simulink model "TestingModels"  (R2021b)
settings: Solver=VariableStepAuto  StartTime=0.0  StopTime=120  FixedStep=1  RelTol=1e-3
libraries: simulink x1
settings Model: Creator=mariodelossantos  LastModifiedBy=mdls3

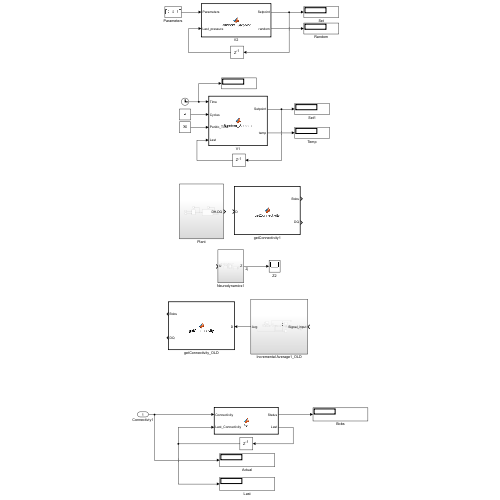
[thumbnail: Simulink's stored preview of the top-level diagram]
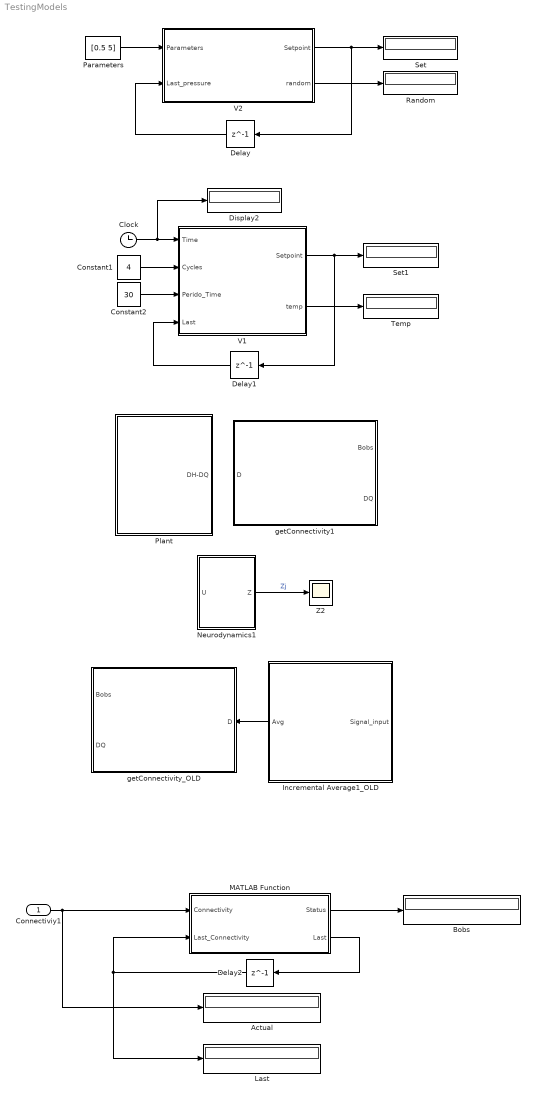
== system TestingModels ==
  Connectiviy1 : Inport
  Actual : Display
  Bobs : Display
  Clock : Clock
  Constant1 : Constant  Value=4
  Constant2 : Constant  Value=30
  Delay : Delay  DelayLength=1  InitialCondition=0
  Delay1 : Delay  DelayLength=1  InitialCondition=0
  Delay2 : Delay  DelayLength=1  InitialCondition=0
  Display2 : Display
  Incremental Average1_OLD : Subsystem
  Last : Display
  MATLAB Function : MATLAB Function  TreatAsAtomicUnit=on
  Neurodynamics1 : Subsystem
  Parameters : Constant  Value=[0.5 5]
  Plant : Subsystem
  Random : Display
  Set : Display
  Set1 : Display
  Temp : Display
  V1 : MATLAB Function  TreatAsAtomicUnit=on
  V2 : MATLAB Function  TreatAsAtomicUnit=on
  Z2 : Scope
  getConnectivity1 : MATLAB Function  TreatAsAtomicUnit=on  SystemSampleTime=0
  getConnectivity_OLD : MATLAB Function  TreatAsAtomicUnit=on  SystemSampleTime=0
  wires:
  Delay/1 -> V2/2(Last_pressure)
  Parameters/1 -> V2/1(Parameters)
  V2/1(Setpoint) -> Delay/1, Set/1
  V2/2(random) -> Random/1
  V1/1(Setpoint) -> Delay1/1, Set1/1
  Delay1/1 -> V1/4(Last)
  Constant1/1 -> V1/2(Cycles)
  Clock/1 -> Display2/1, V1/1(Time)
  Constant2/1 -> V1/3(Perido_Time)
  V1/2(temp) -> Temp/1
  Neurodynamics1/1(Z) -> Z2/1  "Zj"
  Incremental Average1_OLD/1(Avg) -> getConnectivity_OLD/1(D)
  Delay2/1 -> Last/1, MATLAB Function/2(Last_Connectivity)
  MATLAB Function/2(Last) -> Delay2/1
  Connectiviy1/1 -> Actual/1, MATLAB Function/1(Connectivity)
  MATLAB Function/1(Status) -> Bobs/1

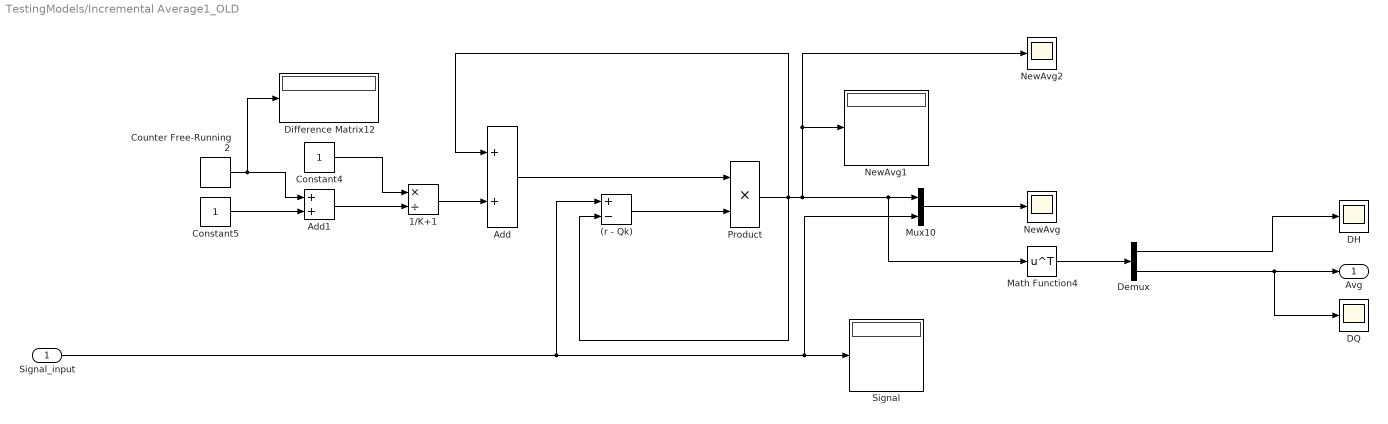
== system TestingModels/Incremental Average1_OLD ==
  Signal_input : Inport
  (r - Qk) : Sum  Inputs=+-
  1/K+1 : Product  Inputs=*/
  Add : Sum
  Add1 : Sum
  Constant4 : Constant
  Constant5 : Constant
  Counter Free-Running2 : simulink/Sources/Counter Free-Running  NumBits=16  tsamp=-1
  DH : Scope
  DQ : Scope
  Demux : Demux  Outputs=2
  Difference Matrix12 : Display
  Math Function4 : Math  Operator=transpose  SaturateOnIntegerOverflow=on
  Mux10 : Mux  Inputs=2
  NewAvg : Scope
  NewAvg1 : Display
  NewAvg2 : Scope
  Product : Product
  Signal : Display
  Avg : Outport
  wires:
  1/K+1/1 -> Add/2
  Counter Free-Running2/1 -> Difference Matrix12/1, Add1/1
  (r - Qk)/1 -> Product/2
  Signal_input/1 -> Mux10/2, Signal/1, (r - Qk)/1
  Add/1 -> Product/1
  Mux10/1 -> NewAvg/1
  Product/1 -> Add/1, (r - Qk)/2, NewAvg2/1, NewAvg1/1, Math Function4/1, Mux10/1
  Add1/1 -> 1/K+1/2
  Constant5/1 -> Add1/2
  Constant4/1 -> 1/K+1/1
  Math Function4/1 -> Demux/1
  Demux/2 -> Avg/1, DQ/1
  Demux/1 -> DH/1

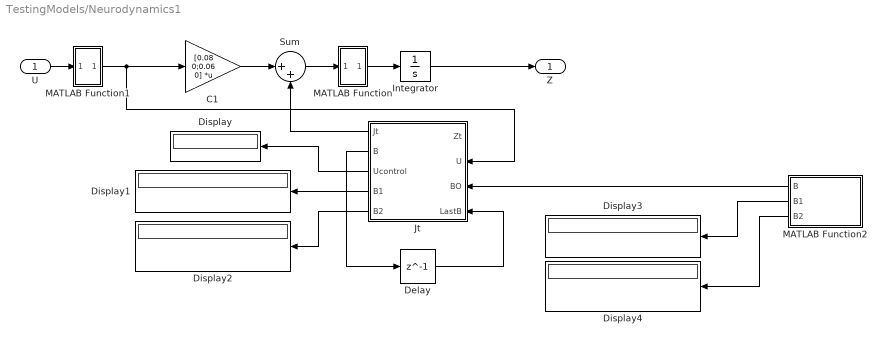
== system TestingModels/Neurodynamics1 ==
  U : Inport
  C1 : Gain  Gain=[0.08 0;0.06 0]  Multiplication=Matrix(K*u) (u vector)
  Delay : Delay  DelayLength=1  InitialCondition=[1 1;1 1]
  Display{,1..4} (5 alike) : Display
  Integrator : Integrator
  Jt : MATLAB Function  TreatAsAtomicUnit=on
  MATLAB Function : MATLAB Function  TreatAsAtomicUnit=on
  MATLAB Function1 : MATLAB Function  TreatAsAtomicUnit=on
  MATLAB Function2 : MATLAB Function  TreatAsAtomicUnit=on
  Sum : Sum  Inputs=|++
  Z : Outport
  wires:
  Integrator/1 -> Z/1
  C1/1 -> Sum/1
  U/1 -> MATLAB Function1/1(Z)
  Sum/1 -> MATLAB Function/1(Z)
  MATLAB Function1/1(Zn) -> C1/1, Jt/2(U)
  MATLAB Function/1(Zn) -> Integrator/1
  Jt/2(B) -> Delay/1
  Jt/3(Ucontrol) -> Display/1
  MATLAB Function2/1(B) -> Jt/3(BO)
  Jt/4(B1) -> Display1/1
  Jt/5(B2) -> Display2/1
  MATLAB Function2/2(B1) -> Display3/1
  MATLAB Function2/3(B2) -> Display4/1
  Delay/1 -> Jt/4(LastB)
  Jt/1(Jt) -> Sum/2

== system TestingModels/Plant ==
  Human Agent : Subsystem
  Period Time U3 : Constant  Value=30
  Period Time U4 : Constant  Value=30
  Stimulus : Scope
  Variable Stimulus1 : Subsystem
  fNIRS : Scope
  DH-DQ : Outport
  wires:
  Human Agent/1(fNIRS) -> fNIRS/1
  Period Time U3/1 -> Variable Stimulus1/1(In1)
  Period Time U4/1 -> Variable Stimulus1/2(In2)
  Human Agent/2(DH-DQ) -> DH-DQ/1
  Variable Stimulus1/1(U) -> Stimulus/1, Human Agent/1(Stimulus)

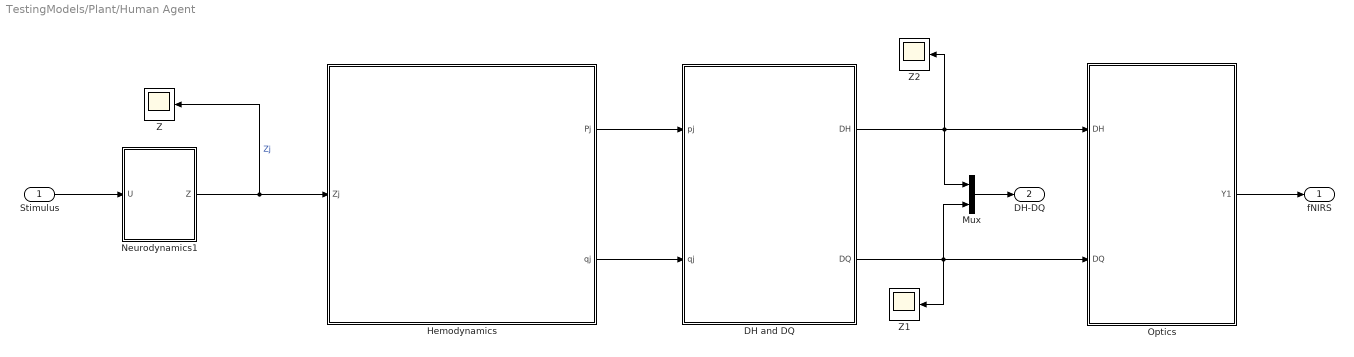
== system TestingModels/Plant/Human Agent ==
  Stimulus : Inport
  DH and DQ : Subsystem
  Hemodynamics : Subsystem
  Mux : Mux  Inputs=2
  Neurodynamics1 : Subsystem
  Optics : Subsystem
  Z : Scope
  Z1 : Scope
  Z2 : Scope
  fNIRS : Outport
  DH-DQ : Outport  Port=2
  wires:
  Hemodynamics/1(Pj) -> DH and DQ/1(pj)
  Hemodynamics/2(qj) -> DH and DQ/2(qj)
  Neurodynamics1/1(Z) -> Z/1, Hemodynamics/1(Zj)  "Zj"
  Stimulus/1 -> Neurodynamics1/1(U)
  DH and DQ/1(DH) -> Z2/1, Mux/1, Optics/1(DH)
  DH and DQ/2(DQ) -> Z1/1, Mux/2, Optics/2(DQ)
  Optics/1(Y1) -> fNIRS/1
  Mux/1 -> DH-DQ/1

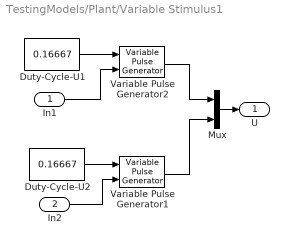
== system TestingModels/Plant/Variable Stimulus1 ==
  In1 : Inport
  In2 : Inport  Port=2
  Duty-Cycle-U1 : Constant  Value=0.16667  OutMin=[0]  OutMax=[0.8]
  Duty-Cycle-U2 : Constant  Value=0.16667  OutMin=[0]  OutMax=[0.8]
  Mux : Mux  Inputs=2
  Variable Pulse Generator1 : VariablePulseGenerator  RunAtFixedTimeIntervals=on  SampleTime=1/100
  Variable Pulse Generator2 : VariablePulseGenerator  RunAtFixedTimeIntervals=on  SampleTime=1/100
  U : Outport
  wires:
  In2/1 -> Variable Pulse Generator1/2
  Mux/1 -> U/1
  Variable Pulse Generator1/1 -> Mux/2
  Duty-Cycle-U2/1 -> Variable Pulse Generator1/1
  In1/1 -> Variable Pulse Generator2/2
  Duty-Cycle-U1/1 -> Variable Pulse Generator2/1
  Variable Pulse Generator2/1 -> Mux/1

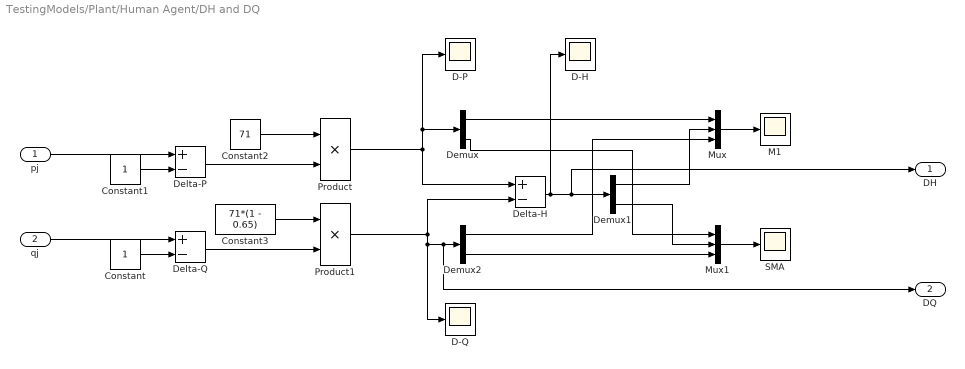
== system TestingModels/Plant/Human Agent/DH and DQ ==
  pj : Inport
  qj : Inport  Port=2
  Constant : Constant
  Constant1 : Constant
  Constant2 : Constant  Value=71
  Constant3 : Constant  Value=71*(1 - 0.65)
  D-H : Scope
  D-P : Scope
  D-Q : Scope
  Delta-H : Sum  Inputs=+-
  Delta-P : Sum  Inputs=+-
  Delta-Q : Sum  Inputs=+-
  Demux : Demux  Outputs=2
  Demux1 : Demux  Outputs=2
  Demux2 : Demux  Outputs=2
  M1 : Scope
  Mux : Mux  Inputs=3
  Mux1 : Mux  Inputs=3
  Product : Product
  Product1 : Product
  SMA : Scope
  DH : Outport
  DQ : Outport  Port=2
  wires:
  Constant2/1 -> Product/1
  Delta-Q/1 -> Product1/2
  Constant3/1 -> Product1/1
  Demux2/2 -> Mux1/3
  pj/1 -> Delta-P/1
  Mux1/1 -> SMA/1
  Demux/2 -> Mux1/1
  Mux/1 -> M1/1
  Constant/1 -> Delta-Q/2
  Delta-P/1 -> Product/2
  Product1/1 -> DQ/1, Demux2/1, D-Q/1, Delta-H/2
  qj/1 -> Delta-Q/1
  Demux/1 -> Mux/1
  Delta-H/1 -> DH/1, Demux1/1, D-H/1
  Demux1/1 -> Mux/2
  Demux1/2 -> Mux1/2
  Product/1 -> Demux/1, D-P/1, Delta-H/1
  Demux2/1 -> Mux/3
  Constant1/1 -> Delta-P/2

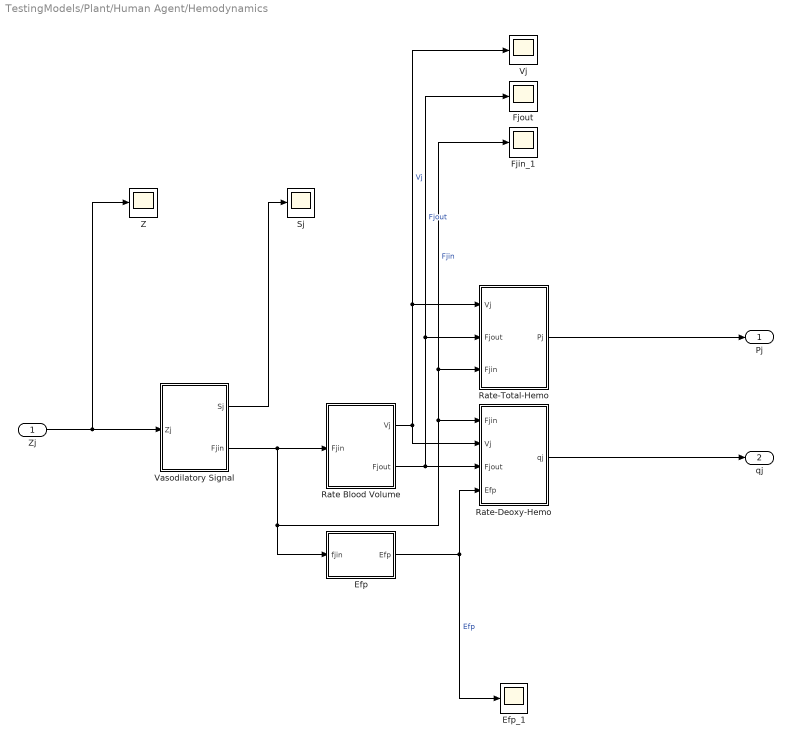
== system TestingModels/Plant/Human Agent/Hemodynamics ==
  Zj : Inport
  Efp : MATLAB Function  TreatAsAtomicUnit=on
  Efp_1 : Scope
  Fjin_1 : Scope
  Fjout : Scope
  Rate Blood Volume : Subsystem
  Rate-Deoxy-Hemo : Subsystem
  Rate-Total-Hemo : Subsystem
  Sj : Scope
  Vasodilatory Signal : Subsystem
  Vj : Scope
  Z : Scope
  Pj : Outport
  qj : Outport  Port=2
  wires:
  Rate-Deoxy-Hemo/1(qj) -> qj/1
  Zj/1 -> Vasodilatory Signal/1(Zj), Z/1
  Vasodilatory Signal/1(Sj) -> Sj/1
  Rate Blood Volume/2(Fjout) -> Fjout/1, Rate-Total-Hemo/2(Fjout), Rate-Deoxy-Hemo/3(Fjout)  "Fjout"
  Rate Blood Volume/1(Vj) -> Vj/1, Rate-Total-Hemo/1(Vj), Rate-Deoxy-Hemo/2(Vj)  "Vj"
  Rate-Total-Hemo/1(Pj) -> Pj/1
  Efp/1(Efp) -> Rate-Deoxy-Hemo/4(Efp), Efp_1/1  "Efp"
  Vasodilatory Signal/2(Fjin) -> Efp/1(fjin), Fjin_1/1, Rate-Total-Hemo/3(Fjin), Rate-Deoxy-Hemo/1(Fjin), Rate Blood Volume/1(Fjin)  "Fjin"

== system TestingModels/Plant/Human Agent/Neurodynamics1 ==
  U : Inport
  C : Gain  Gain=[0.08 0;0.06 0]  Multiplication=Matrix(K*u)
  Integrator : Integrator
  Jt : MATLAB Function  TreatAsAtomicUnit=on
  Sum : Sum  Inputs=|++
  Z : Outport
  wires:
  Integrator/1 -> Z/1, Jt/1(Zt)
  C/1 -> Sum/1
  Jt/1(Jt) -> Sum/2
  U/1 -> C/1, Jt/2(U)
  Sum/1 -> Integrator/1

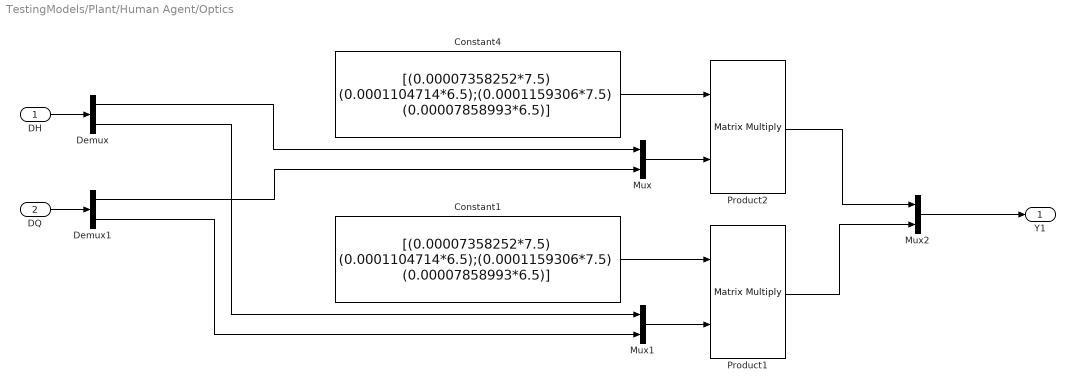
== system TestingModels/Plant/Human Agent/Optics ==
  DH : Inport
  DQ : Inport  Port=2
  Constant1 : Constant  Value=[(0.00007358252*7.5) (0.0001104714*6.5);(0.0001159306*7.5) (0.00007858993*6.5)]
  Constant4 : Constant  Value=[(0.00007358252*7.5) (0.0001104714*6.5);(0.0001159306*7.5) (0.00007858993*6.5)]
  Demux : Demux  Outputs=2
  Demux1 : Demux  Outputs=2
  Mux : Mux  Inputs=2
  Mux1 : Mux  Inputs=2
  Mux2 : Mux  Inputs=2
  Product1 : Product  Multiplication=Matrix(*)
  Product2 : Product  Multiplication=Matrix(*)
  Y1 : Outport
  wires:
  Mux/1 -> Product2/2
  Product2/1 -> Mux2/1
  Mux1/1 -> Product1/2
  Product1/1 -> Mux2/2
  Constant1/1 -> Product1/1
  DH/1 -> Demux/1
  Demux/1 -> Mux/1
  Demux/2 -> Mux1/1
  DQ/1 -> Demux1/1
  Constant4/1 -> Product2/1
  Demux1/1 -> Mux/2
  Demux1/2 -> Mux1/2
  Mux2/1 -> Y1/1

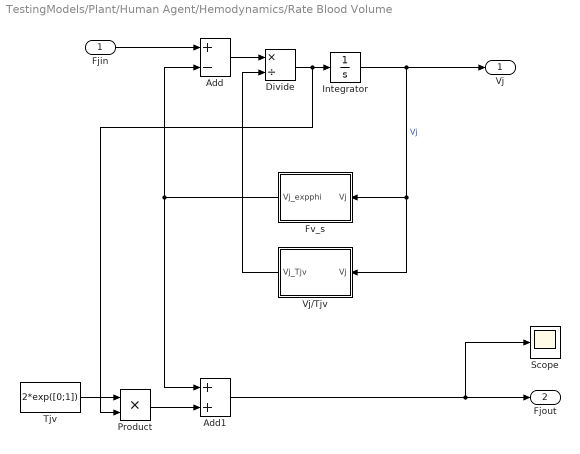
== system TestingModels/Plant/Human Agent/Hemodynamics/Rate Blood Volume ==
  Fjin : Inport
  Add : Sum  Inputs=+-
  Add1 : Sum
  Divide : Product  Inputs=*/
  Fv_s : MATLAB Function  TreatAsAtomicUnit=on
  Integrator : Integrator  InitialCondition=exp([0;0])
  Product : Product
  Scope : Scope
  Tjv : Constant  Value=2*exp([0;1])
  Vj/Tjv : MATLAB Function  TreatAsAtomicUnit=on
  Vj : Outport
  Fjout : Outport  Port=2
  wires:
  Fjin/1 -> Add/1
  Integrator/1 -> Vj/1, Vj/Tjv/1(Vj), Fv_s/1(Vj)  "Vj"
  Divide/1 -> Product/2, Integrator/1
  Fv_s/1(Vj_expphi) -> Add/2, Add1/1
  Add/1 -> Divide/1
  Vj/Tjv/1(Vj_Tjv) -> Divide/2
  Product/1 -> Add1/2
  Tjv/1 -> Product/1
  Add1/1 -> Scope/1, Fjout/1

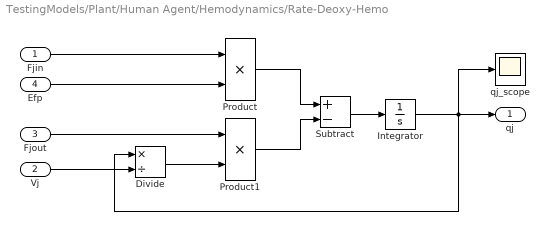
== system TestingModels/Plant/Human Agent/Hemodynamics/Rate-Deoxy-Hemo ==
  Fjin : Inport
  Vj : Inport  Port=2
  Fjout : Inport  Port=3
  Efp : Inport  Port=4
  Divide : Product  Inputs=*/
  Integrator : Integrator  InitialCondition=exp([0;0])
  Product : Product
  Product1 : Product
  Subtract : Sum  Inputs=+-
  qj_scope : Scope
  qj : Outport
  wires:
  Efp/1 -> Product/2
  Divide/1 -> Product1/2
  Subtract/1 -> Integrator/1
  Integrator/1 -> qj/1, Divide/1, qj_scope/1
  Vj/1 -> Divide/2
  Product1/1 -> Subtract/2
  Fjin/1 -> Product/1
  Fjout/1 -> Product1/1
  Product/1 -> Subtract/1

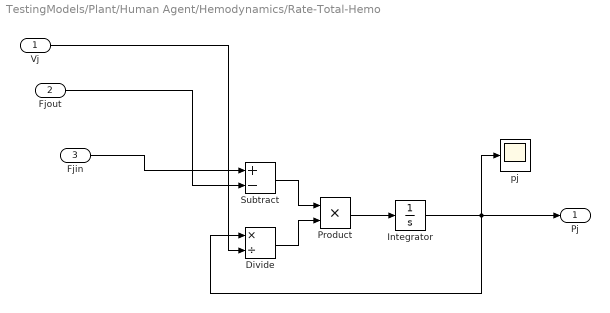
== system TestingModels/Plant/Human Agent/Hemodynamics/Rate-Total-Hemo ==
  Vj : Inport
  Fjout : Inport  Port=2
  Fjin : Inport  Port=3
  Divide : Product  Inputs=*/
  Integrator : Integrator  InitialCondition=exp([0;0])
  Product : Product
  Subtract : Sum  Inputs=+-
  pj : Scope
  Pj : Outport
  wires:
  Fjout/1 -> Subtract/2
  Product/1 -> Integrator/1
  Vj/1 -> Divide/2
  Subtract/1 -> Product/1
  Fjin/1 -> Subtract/1
  Divide/1 -> Product/2
  Integrator/1 -> Pj/1, pj/1, Divide/1

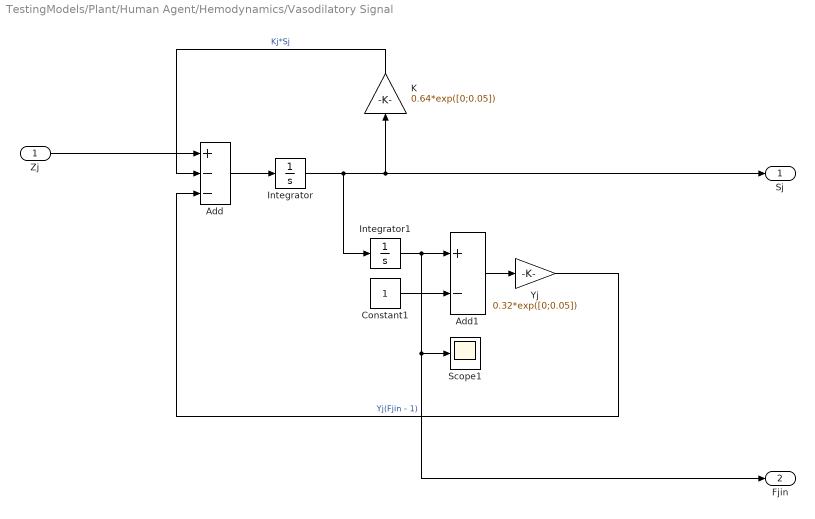
== system TestingModels/Plant/Human Agent/Hemodynamics/Vasodilatory Signal ==
  Zj : Inport
  Add : Sum  Inputs=+--
  Add1 : Sum  Inputs=+-
  Constant1 : Constant
  Integrator : Integrator
  Integrator1 : Integrator  InitialCondition=exp([0;0])
  K : Gain  Gain=0.64*exp([0;0.05])
  Scope1 : Scope
  Yj : Gain  Gain=0.32*exp([0;0.05])
  Sj : Outport
  Fjin : Outport  Port=2
  wires:
  Add1/1 -> Yj/1
  K/1 -> Add/2  "Kj*Sj"
  Constant1/1 -> Add1/2
  Zj/1 -> Add/1
  Integrator1/1 -> Fjin/1, Scope1/1, Add1/1
  Integrator/1 -> Sj/1, K/1, Integrator1/1
  Add/1 -> Integrator/1
  Yj/1 -> Add/3  "Yj(Fjin - 1)"

== matlab function TestingModels/MATLAB Function ==
  data: Connectivity input; Status output; Last_Connectivity input; Last output
function [Status, Last] = fcn(Connectivity, Last_Connectivity)
temp = 0;
if Connectivity(:,:) ~= Last_Connectivity(:,:)
    temp = 1;
else
    temp = 0;
end 

Status  = temp;
Last = Connectivity;

== matlab function TestingModels/Plant/Human Agent/Hemodynamics/Rate Blood Volume/Fv_s ==
  data: Vj input; Vj_expphi output
function Vj_expphi = fcn(Vj)
phi = 0.32;
Vj_expphi = Vj.^(1/phi);

== matlab function TestingModels/getConnectivity_OLD ==
  data: D input; Bobs output; DQ output
function [Bobs, DQ] = getConnectivity(D)

    DQ = [nan;nan];
    DQ(1) = D(1);
    DQ(2) = D(2);

    rThresh= 0.6; % [0..1] A threshold on the correlation.

    [nSamples, nChannels, nHb]=size(D);

    C = nan(nChannels, nChannels, nHb); %Matrix of channel pairwise correlations;

    %This part of the algorithm is HIGHLY inefficient but it does the job for now
    %but might not be sufficiently fast for "real time" neurofeedback

    for iHb = 1:nHb
        for iCh=1:nChannels
            for jCh=iCh:nChannels

                if iCh == jCh

                 C(iCh,jCh,iHb) = 1;

               else

                 C(iCh,jCh,iHb) = xcorr2(D(:,iCh,iHb),D(:,jCh,iHb));

                end
            end

        end

    end

    %Threshold/Binarize C

    tmp = C > rThresh;

    %Finally "merge" accross Hb species

    Bobs = all(tmp,3); %Apply the AND function across Hb species.

== matlab function TestingModels/V1 ==
  settings: updateMethod=DISCRETE
  data: Setpoint output; Time input; Cycles input; Perido_Time input; Last input; temp output
function [Setpoint, temp] = Random_Setpoint(Time, Cycles,Perido_Time, Last)
    Pcycles = ones(Cycles);
    temp = 0;
    min = 0;
    max = 8;
    r = min + rand(1)*(max-min);
    for i = 1:Cycles
        Pcycles(i) = i;
        Pcycles(i) = i*Perido_Time;
        %We should fine a random criteria to change the setpoint, not just
        %time, or the moment B changes. For now works to demostrate the
        %control without fNIRS
         if (Time > (Pcycles(i)-0.5)) && (Time < (Pcycles(i)+1))
            %disp("Time")
            %disp(Time)
            temp = r;
            %disp("Setpoint")
            %disp(temp)
        else 
            temp = Last;
        end  
    end

    Setpoint = temp;

== matlab function TestingModels/Neurodynamics1/Jt ==
  settings: updateMethod=DISCRETE
  data: Zt input; U input; BO input; Jt output; B output; Ucontrol output; B1 output; B2 output; LastB input
function [Jt, B, Ucontrol, B1,B2] = fcn(Zt, U, BO, LastB)
   Bt = zeros(2,2,2);

   none = ones(2,2);
   if LastB == none
       LastB = BO;
   else
       LastB = LastB;
   end

   A = [-0.16 -0.49;-0.02 -0.33];
   threshold = 0.2;
   nRegions  = size(A,1);
   M = size(U,1); %nStimuli
   simulationLength = size(U,2);

   Weight_U = 0 + rand(1)*(1);
   Ucontrol = U(2) * Weight_U;
   
      assert(M == size(BO,3),...
       'Unexpected number of induced connectivity parameters B.');

   T = zeros(nRegions); %nRegions x nRegions

    for t = 1:simulationLength
           if Ucontrol < threshold
                min = -2; 
                max = 2;
                n = nRegions;
                r1 = min + rand(n)*(max-min);
                r2 = min + rand(n)*(max-min);
                Bt(:,:,1) = r1(:,:);
                Bt(:,:,2) = r2(:,:);
           else
               Bt = LastB;
   
           end
           B = Bt;

           for uu = 1:M % Sum (Uj * Bj)
               tmp = U(uu,t)*B(:,:,uu);
               T = -0.5*exp(T + tmp);  
           end

     
    end
    
    SI = diag(A);
    A =  A - diag(exp(SI) + (SI));

B1 = B(:,:,1);   
B2 = B(:,:,2);  
Jt = (A*Zt) + (T*Zt);

== matlab function TestingModels/V2 ==
  settings: updateMethod=DISCRETE
  data: Setpoint output; Parameters input; Last_pressure input; random output
function [Setpoint, random] = Random_Setpoint(Parameters, Last_pressure)


    %Parameters = [threshold Start_setpoint]

    %Random used to simulate the connectivity changes, so we must change
    %the pressure setpoint when changes in the connectitvy are observed.
    tmin = 0;
    tmax = 5;
        %We should fine a random criteria to change the setpoint, not just
        %time, or the moment B changes. For now works to demostrate the
        %control without fNIRS
    random = tmin + rand(1) * (tmax - tmin);

    temp = 0;
   %Pressure Setpoint selection
    pmin = 0;
    pmax = 8;
    new_pressure = pmin + rand(1)*(pmax-pmin);
         if (random < Parameters(1))
            %disp("Time")
            %disp(Time)
            temp = new_pressure;
            %disp("Setpoint")
            %disp(temp)
        else 
            temp = Last_pressure;
                if (Parameters(2) == temp || temp == 0)
                    temp = Parameters(2);
                else
                    temp = Last_pressure;
                end
        end  

    Setpoint = temp;

== matlab function TestingModels/Plant/Human Agent/Hemodynamics/Efp ==
  data: fjin input; Efp output
function Efp= fcn(fjin)

Efp = (1 - (1 - 0.32).^ (1 ./ fjin))/0.32;

== matlab function TestingModels/Plant/Human Agent/Hemodynamics/Rate Blood Volume/Vj//Tjv ==
  data: Vj input; Vj_Tjv output
function Vj_Tjv = fcn(Vj)
    Tjv = 2*exp([0;1]);
    Tj = 2*exp([0;0.05]);
Vj_Tjv =(Tj.*Tjv.*Vj);

== matlab function TestingModels/Neurodynamics1/MATLAB Function ==
  data: Z input; Zn output
function Zn = fcn(Z)

Zn = Z(:,1);

== matlab function TestingModels/Neurodynamics1/MATLAB Function1 ==
  data: Z input; Zn output
function Zn = fcn(Z)

Zn = Z(:,1);

== matlab function TestingModels/Neurodynamics1/MATLAB Function2 ==
  data: B output; B1 output; B2 output
function [B, B1, B2] = B() 
   B = zeros(2,2,2);
   B1 = [0 0; 0 0]; %There must be a B per stimulus
   B2 = [-0.02 -0.77; 0.33 -1.31];
   B(:,:,1) = B1;
   B(:,:,2) = B2;

== matlab function TestingModels/Plant/Human Agent/Neurodynamics1/Jt ==
  data: Zt input; U input; Jt output
function Jt = fcn(Zt, U)
   A = [-0.16 -0.49;-0.02 -0.33];
   nRegions  = size(A,1);
   M = size(U,1); %nStimuli
   simulationLength = size(U,2);
   B = zeros(2,2,2);
   B1 = [0 0; 0 0]; %There must be a B per stimulus
   B2 = [-0.02 -0.77; 0.33 -1.31];
   B(:,:,1) = B1;
   B(:,:,2) = B2;
      assert(M == size(B,3),...
       'Unexpected number of induced connectivity parameters B.');
   T = zeros(nRegions); %nRegions x nRegions
    for t = 1:simulationLength
           for uu = 1:M % Sum (Uj * Bj)
               tmp = U(uu,t)*B(:,:,uu);
               T = -0.5*exp(T + tmp);  
           end
    end
    SI = diag(A);
    A =  A - diag(exp(SI) + (SI));
Jt = (A*Zt) + (T*Zt);

== matlab function TestingModels/getConnectivity1 ==
  data: D input; Bobs output; DQ output
function [Bobs, DQ] = getConnectivity(D)

    DQ = [nan;nan];
    DQ(1) = D(1);
    DQ(2) = D(2);

    rThresh= 0.6; % [0..1] A threshold on the correlation.

    [nSamples, nChannels, nHb] = size(D);

    C = nan(nChannels, nChannels, nHb); %Matrix of channel pairwise correlations;

    %This part of the algorithm is HIGHLY inefficient but it does the job for now
    %but might not be sufficiently fast for "real time" neurofeedback

    for iHb = 1:nHb
        for iCh=1:nChannels
            for jCh=iCh:nChannels

                if iCh == jCh

                 C(iCh,jCh,iHb) = 1;

               else

                 C(iCh,jCh,iHb) = xcorr2(D(:,iCh,iHb),D(:,jCh,iHb));

                end
            end

        end

    end

    %Threshold/Binarize C

    tmp = C > rThresh;

    %Finally "merge" accross Hb species

    Bobs = all(tmp,3); %Apply the AND function across Hb species.
